simulink model "FG_traj"  (Simulink 7.8)
settings: Solver=FixedStepDiscrete  StartTime=0.0  StopTime=inf  FixedStep=Ts  RelTol=1e-3
PreLoadFcn:
  | load_waypoints
values from neighbouring files (symbols this model uses):
  g = 9.8065    [kostas_malakies.mat]    (also in kostas_malakies2.mat; load_PMModel.m = 9.81; main.m; main_last.m)
  mass = 0.66    [kostas_malakies.mat]    (also in kostas_malakies2.mat; load_PMModel.m = 0.687; main_last.m)
  pitch_cmd2pitch_1stOrd = 1.42468924998    [kostas_malakies.mat]    (also in kostas_malakies2.mat)
  roll_cmd2roll_1stOrd = 1.38101661575    [kostas_malakies.mat]    (also in kostas_malakies2.mat)
  thrust_cmd2thrust_0thOrd = 0.876575459522    [kostas_malakies.mat]    (also in kostas_malakies2.mat)
  THRUST_CMD_GAIN = -0.0835    [kostas_malakies.mat]    (also in kostas_malakies2.mat; load_PMModel.m)
  Ts = 0.02    [kostas_malakies.mat]    (also in kostas_malakies2.mat; main.m; main_last.m; matlab.mat = 0.08)
  yaw_cmd2yaw_1stOrd = 2.01792090263    [kostas_malakies.mat]    (also in kostas_malakies2.mat)
undefined symbols (not defined in the file or in its folder): DiscIntNeverNeededParam
libraries: Hquad_control_LIB_MPC x22, simulink x2
settings Model: Creator=janosch  LastModifiedBy=burrimi  SimulationMode=external
settings DataIOCC: SaveOutput=off  SaveTime=off
settings OptimizationCC: OptimizeModelRefInitCode=on  LifeSpan=Inf
settings DebuggingCC: ParameterPrecisionLossMsg=none  FcnCallInpInsideContextMsg=Use local settings
settings HardwareCC: ProdIntDivRoundTo=Zero  ProdEndianess=LittleEndian  ProdHWDeviceType=Intel Pentium
settings RTWCC: SystemTargetFile=ert.tlc  TemplateMakefile=ert_default_tmf  Description=Embedded Coder  ProcessScript=ert_make_rtw_hook  CustomHeaderCode=#include <math.h>  TargetLang=C++
settings CodeAppCC: IgnoreCustomStorageClasses=off
settings ERTTargetCC: MultiwordLength=2048  GenerateSampleERTMain=on  ExtMode=on  ERTCustomFileTemplate=example_file_process.tlc  ConvertIfToSwitch=off  SuppressUnreachableDefaultCases=off

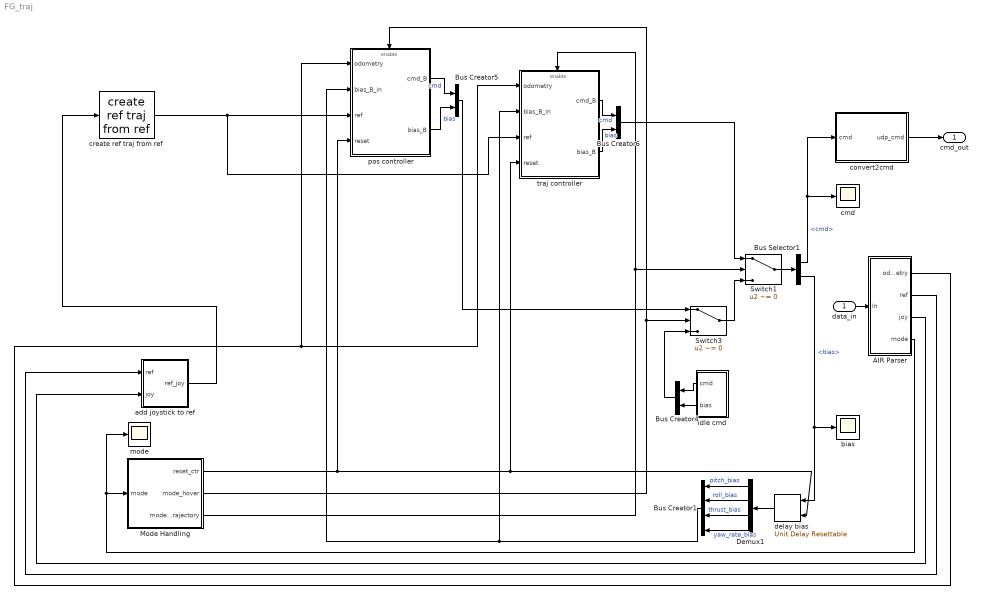
== system FG_traj ==
  data_in : Inport  OutDataTypeStr=single  PortDimensions=30
  AIR Parser : Subsystem
  Bus Creator1 : BusCreator
  Bus Creator4 : BusCreator  Inputs=2
  Bus Creator5 : BusCreator  Inputs=2
  Bus Creator6 : BusCreator  Inputs=2
  Bus Selector1 : BusSelector  OutputSignals=cmd,bias
  Demux1 : Demux
  Idle cmd : Subsystem
  Mode Handling : Subsystem
  Switch1 : Switch  Criteria=u2 ~= 0
  Switch3 : Switch  Criteria=u2 ~= 0
  add joystick to ref : Subsystem
  bias : Scope
      settings: TickLabels=on  TimeRange=40  YMin=-0.3  YMax=0.075  SaveName=ScopeData9
  cmd : Scope
      settings: YMin=-0.5  YMax=7  SaveName=ScopeData4
  convert2cmd : Subsystem
  create ref traj from ref : Hquad_control_LIB_MPC/create ref traj from ref
  delay bias : simulink/Additional Math & Discrete/Additional Discrete/Unit Delay Resettable  vinit=0.0  tsamp=-1
  mode : Scope
      settings: YMin=0  YMax=6  SaveName=ScopeData6
  pos controller : Subsystem  AncestorBlock=Hquad_control_LIB_MPC/pos controller
  traj controller : Subsystem  AncestorBlock=Hquad_control_LIB_MPC/traj controller
  cmd_out : Outport  PortDimensions=4
  wires:
  Mode Handling/1(reset_ctr) -> delay bias/2, traj controller/4(reset), pos controller/4(reset)
  Mode Handling/2(mode_hover) -> Switch3/2, pos controller/Enable
  Mode Handling/3(mode_trajectory) -> Switch1/2, traj controller/Enable
  Switch3/1 -> Switch1/3
  AIR Parser/3(joy) -> add joystick to ref/2(joy)
  add joystick to ref/1(ref_joy) -> create ref traj from ref/1
  AIR Parser/2(ref) -> add joystick to ref/1(ref)
  AIR Parser/1(odometry) -> pos controller/1(odometry), traj controller/1(odometry)
  AIR Parser/4(mode) -> Mode Handling/1(mode), mode/1
  create ref traj from ref/1 -> pos controller/3(ref), traj controller/3(ref)
  Idle cmd/1(cmd) -> Bus Creator4/1
  Idle cmd/2(bias) -> Bus Creator4/2
  Bus Creator4/1 -> Switch3/3
  traj controller/1(cmd_B) -> Bus Creator6/1  "cmd"
  traj controller/2(bias_B) -> Bus Creator6/2  "bias"
  Bus Creator6/1 -> Switch1/1
  Bus Creator5/1 -> Switch3/1
  pos controller/1(cmd_B) -> Bus Creator5/1  "cmd"
  pos controller/2(bias_B) -> Bus Creator5/2  "bias"
  Switch1/1 -> Bus Selector1/1
  Bus Selector1/1 -> cmd/1, convert2cmd/1(cmd)  "<cmd>"
  Bus Selector1/2 -> delay bias/1, bias/1  "<bias>"
  Demux1/1 -> Bus Creator1/1  "pitch_bias"
  Demux1/2 -> Bus Creator1/2  "roll_bias"
  Demux1/3 -> Bus Creator1/3  "thrust_bias"
  Demux1/4 -> Bus Creator1/4  "yaw_rate_bias"
  delay bias/1 -> Demux1/1
  Bus Creator1/1 -> pos controller/2(bias_B_in), traj controller/2(bias_B_in)
  convert2cmd/1(udp_cmd) -> cmd_out/1
  data_in/1 -> AIR Parser/1(In)

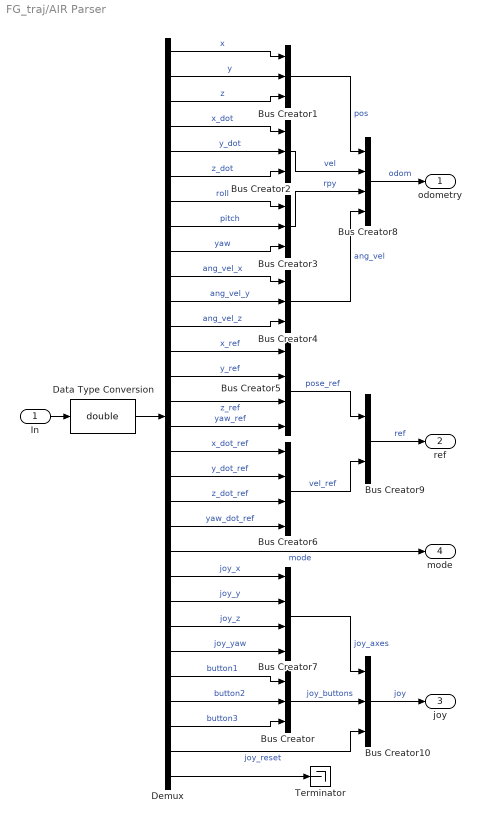
== system FG_traj/AIR Parser ==
  In : Inport
  Bus Creator{,1..4,10} (6 alike) : BusCreator  Inputs=3
  Bus Creator{5..8} (4 alike) : BusCreator
  Bus Creator9 : BusCreator  Inputs=2
  Data Type Conversion : DataTypeConversion  OutDataTypeStr=double
  Demux : Demux  Outputs=30
  Terminator : Terminator
  odometry : Outport
  ref : Outport  Port=2
  joy : Outport  Port=3
  mode : Outport  Port=4
  wires:
  In/1 -> Data Type Conversion/1
  Data Type Conversion/1 -> Demux/1
  Demux/1 -> Bus Creator1/1  "x"
  Demux/7 -> Bus Creator3/1  "roll"
  Demux/8 -> Bus Creator3/2  "pitch"
  Demux/9 -> Bus Creator3/3  "yaw"
  Demux/15 -> Bus Creator5/3  "z_ref"
  Demux/14 -> Bus Creator5/2  "y_ref"
  Demux/13 -> Bus Creator5/1  "x_ref"
  Demux/16 -> Bus Creator5/4  "yaw_ref"
  Demux/2 -> Bus Creator1/2  "y"
  Demux/3 -> Bus Creator1/3  "z"
  Demux/4 -> Bus Creator2/1  "x_dot"
  Demux/5 -> Bus Creator2/2  "y_dot"
  Demux/6 -> Bus Creator2/3  "z_dot"
  Demux/19 -> Bus Creator6/3  "z_dot_ref"
  Demux/18 -> Bus Creator6/2  "y_dot_ref"
  Demux/17 -> Bus Creator6/1  "x_dot_ref"
  Demux/20 -> Bus Creator6/4  "yaw_dot_ref"
  Demux/12 -> Bus Creator4/3  "ang_vel_z"
  Demux/11 -> Bus Creator4/2  "ang_vel_y"
  Demux/10 -> Bus Creator4/1  "ang_vel_x"
  Demux/21 -> mode/1  "mode"
  Bus Creator5/1 -> Bus Creator9/1  "pose_ref"
  Bus Creator6/1 -> Bus Creator9/2  "vel_ref"
  Demux/22 -> Bus Creator7/1  "joy_x"
  Demux/23 -> Bus Creator7/2  "joy_y"
  Demux/24 -> Bus Creator7/3  "joy_z"
  Demux/25 -> Bus Creator7/4  "joy_yaw"
  Bus Creator7/1 -> Bus Creator10/1  "joy_axes"
  Demux/26 -> Bus Creator/1  "button1"
  Demux/28 -> Bus Creator/3  "button3"
  Demux/27 -> Bus Creator/2  "button2"
  Bus Creator/1 -> Bus Creator10/2  "joy_buttons"
  Bus Creator4/1 -> Bus Creator8/4  "ang_vel"
  Bus Creator3/1 -> Bus Creator8/3  "rpy"
  Bus Creator2/1 -> Bus Creator8/2  "vel"
  Bus Creator1/1 -> Bus Creator8/1  "pos"
  Demux/29 -> Bus Creator10/3  "joy_reset"
  Bus Creator10/1 -> joy/1  "joy"
  Bus Creator9/1 -> ref/1  "ref"
  Bus Creator8/1 -> odometry/1  "odom"
  Demux/30 -> Terminator/1

== system FG_traj/Idle cmd ==
  Bus Creator : BusCreator
  Bus Creator3 : BusCreator
  pitch : Constant  Value=0
  pitch_bias : Constant  Value=0
  roll : Constant  Value=0
  roll_bias : Constant  Value=0
  thrust : Constant  Value=-mass*g
  thrust_bias : Constant  Value=0
  yaw : Constant  Value=0
  yaw_rate_bias : Constant  Value=0
  cmd : Outport
  bias : Outport  Port=2
  wires:
  roll/1 -> Bus Creator/2  "roll_cmd"
  pitch/1 -> Bus Creator/1  "pitch_cmd"
  Bus Creator/1 -> cmd/1  "cmd"
  thrust/1 -> Bus Creator/3  "thrust_cmd"
  yaw/1 -> Bus Creator/4  "yaw_rate_cmd"
  pitch_bias/1 -> Bus Creator3/1  "pitch_bias"
  roll_bias/1 -> Bus Creator3/2  "roll_bias"
  thrust_bias/1 -> Bus Creator3/3  "thrust_bias"
  yaw_rate_bias/1 -> Bus Creator3/4  "yaw_rate_bias"
  Bus Creator3/1 -> bias/1  "bias"

== system FG_traj/Mode Handling ==
  mode : Inport
  Constant1 : Constant
  Constant2 : Constant  Value=0
  Multiport Switch : MultiPortSwitch  DataPortOrder=Specify indices  Inputs=2  DataPortIndices={[1,2,3],0}  zeroidx=off
  Multiport Switch1 : MultiPortSwitch  DataPortOrder=Specify indices  Inputs=2  DataPortIndices={[10],0}  zeroidx=off
  Multiport Switch2 : MultiPortSwitch  DataPortOrder=Specify indices  Inputs=2  DataPortIndices={[4],0}  zeroidx=off
  reset_ctr : Outport
  mode_hover : Outport  Port=2
  mode_trajectory : Outport  Port=3
  wires:
  Constant1/1 -> Multiport Switch/2, Multiport Switch1/2, Multiport Switch2/2
  Constant2/1 -> Multiport Switch/3, Multiport Switch1/3, Multiport Switch2/3
  Multiport Switch1/1 -> reset_ctr/1
  mode/1 -> Multiport Switch/1, Multiport Switch1/1, Multiport Switch2/1
  Multiport Switch/1 -> mode_hover/1
  Multiport Switch2/1 -> mode_trajectory/1

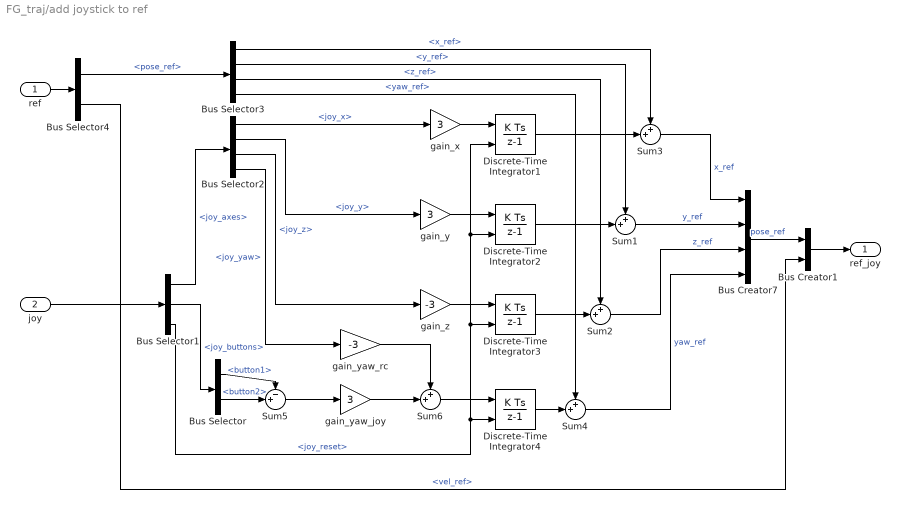
== system FG_traj/add joystick to ref ==
  ref : Inport
  joy : Inport  Port=2
  Bus Creator1 : BusCreator  Inputs=2
  Bus Creator7 : BusCreator
  Bus Selector : BusSelector  OutputSignals=button1,button2
  Bus Selector1 : BusSelector  OutputSignals=joy_axes,joy_buttons,joy_reset
  Bus Selector2 : BusSelector  OutputSignals=joy_x,joy_y,joy_z,joy_yaw
  Bus Selector3 : BusSelector  OutputSignals=x_ref,y_ref,z_ref,yaw_ref
  Bus Selector4 : BusSelector  OutputSignals=pose_ref,vel_ref
  Discrete-Time Integrator{1..4} (4 alike) : DiscreteIntegrator  ExternalReset=rising  SampleTime=Ts  ICPrevOutput=DiscIntNeverNeededParam  ICPrevScaledInput=DiscIntNeverNeededParam
  Sum{1..4,6} (5 alike) : Sum  Inputs=++|
  Sum5 : Sum  Inputs=-+|
  gain_x : Gain  Gain=3
  gain_y : Gain  Gain=3
  gain_yaw_joy : Gain  Gain=3
  gain_yaw_rc : Gain  Gain=-3
  gain_z : Gain  Gain=-3
  ref_joy : Outport
  wires:
  Bus Selector2/1 -> gain_x/1  "<joy_x>"
  Bus Selector2/2 -> gain_y/1  "<joy_y>"
  Bus Selector2/3 -> gain_z/1  "<joy_z>"
  gain_x/1 -> Discrete-Time Integrator1/1
  gain_y/1 -> Discrete-Time Integrator2/1
  gain_z/1 -> Discrete-Time Integrator3/1
  Bus Selector3/1 -> Sum3/1  "<x_ref>"
  Bus Selector3/2 -> Sum1/1  "<y_ref>"
  Bus Selector3/3 -> Sum2/1  "<z_ref>"
  Discrete-Time Integrator1/1 -> Sum3/2
  Discrete-Time Integrator2/1 -> Sum1/2
  Discrete-Time Integrator3/1 -> Sum2/2
  Sum4/1 -> Bus Creator7/4  "yaw_ref"
  Sum2/1 -> Bus Creator7/3  "z_ref"
  Sum1/1 -> Bus Creator7/2  "y_ref"
  Sum3/1 -> Bus Creator7/1  "x_ref"
  Bus Selector1/2 -> Bus Selector/1  "<joy_buttons>"
  Bus Selector1/3 -> Discrete-Time Integrator3/2, Discrete-Time Integrator1/2, Discrete-Time Integrator2/2, Discrete-Time Integrator4/2  "<joy_reset>"
  Bus Selector/1 -> Sum5/1  "<button1>"
  Bus Selector/2 -> Sum5/2  "<button2>"
  Discrete-Time Integrator4/1 -> Sum4/2
  Bus Selector3/4 -> Sum4/1  "<yaw_ref>"
  joy/1 -> Bus Selector1/1
  Bus Selector1/1 -> Bus Selector2/1  "<joy_axes>"
  ref/1 -> Bus Selector4/1
  Bus Creator1/1 -> ref_joy/1
  Sum5/1 -> gain_yaw_joy/1
  Sum6/1 -> Discrete-Time Integrator4/1
  Bus Selector2/4 -> gain_yaw_rc/1  "<joy_yaw>"
  gain_yaw_rc/1 -> Sum6/1
  gain_yaw_joy/1 -> Sum6/2
  Bus Creator7/1 -> Bus Creator1/1  "pose_ref"
  Bus Selector4/1 -> Bus Selector3/1  "<pose_ref>"
  Bus Selector4/2 -> Bus Creator1/2  "<vel_ref>"

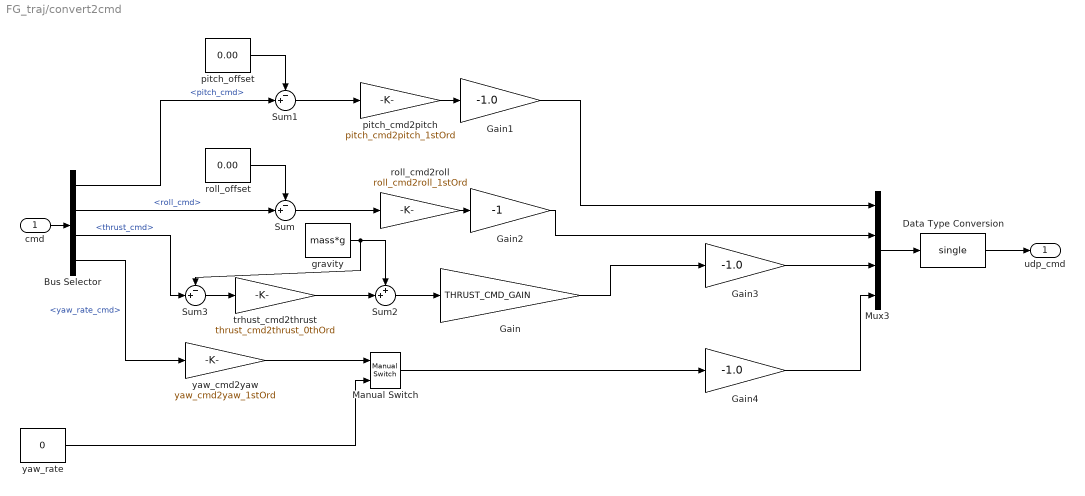
== system FG_traj/convert2cmd ==
  cmd : Inport
  Bus Selector : BusSelector  OutputSignals=pitch_cmd,roll_cmd,thrust_cmd,yaw_rate_cmd
  Data Type Conversion : DataTypeConversion  OutDataTypeStr=single
  Gain : Gain  Gain=THRUST_CMD_GAIN
  Gain1 : Gain  Gain=-1.0
  Gain2 : Gain  Gain=-1
  Gain3 : Gain  Gain=-1.0
  Gain4 : Gain  Gain=-1.0
  Manual Switch : simulink/Signal Routing/Manual Switch  sw=1  action=0  varsize=off
  Mux3 : Mux
  Sum : Sum  Inputs=-+|
  Sum1 : Sum  Inputs=-+|
  Sum2 : Sum  Inputs=++|
  Sum3 : Sum  Inputs=-+|
  gravity : Constant  Value=mass*g
  pitch_cmd2pitch : Gain  Gain=pitch_cmd2pitch_1stOrd
  pitch_offset : Constant  Value=0.00
  roll_cmd2roll : Gain  Gain=roll_cmd2roll_1stOrd
  roll_offset : Constant  Value=0.00
  trhust_cmd2thrust : Gain  Gain=thrust_cmd2thrust_0thOrd
  yaw_cmd2yaw : Gain  Gain=yaw_cmd2yaw_1stOrd
  yaw_rate : Constant  Value=0
  udp_cmd : Outport
  wires:
  pitch_cmd2pitch/1 -> Gain1/1
  Bus Selector/2 -> Sum/2  "<roll_cmd>"
  Sum/1 -> roll_cmd2roll/1
  roll_offset/1 -> Sum/1
  Gain4/1 -> Mux3/4
  Gain3/1 -> Mux3/3
  Gain2/1 -> Mux3/2
  Gain/1 -> Gain3/1
  Gain1/1 -> Mux3/1
  pitch_offset/1 -> Sum1/1
  Sum1/1 -> pitch_cmd2pitch/1
  Mux3/1 -> Data Type Conversion/1
  Data Type Conversion/1 -> udp_cmd/1
  gravity/1 -> Sum2/1, Sum3/1
  Sum2/1 -> Gain/1
  Manual Switch/1 -> Gain4/1
  yaw_rate/1 -> Manual Switch/2
  cmd/1 -> Bus Selector/1
  Bus Selector/1 -> Sum1/2  "<pitch_cmd>"
  yaw_cmd2yaw/1 -> Manual Switch/1
  trhust_cmd2thrust/1 -> Sum2/2
  roll_cmd2roll/1 -> Gain2/1
  Bus Selector/3 -> Sum3/2  "<thrust_cmd>"
  Sum3/1 -> trhust_cmd2thrust/1
  Bus Selector/4 -> yaw_cmd2yaw/1  "<yaw_rate_cmd>"

== system FG_traj/pos controller ==
  odometry : Inport
  bias_B_in : Inport  Port=2
  ref : Inport  Port=3
  reset : Inport  Port=4
  Enable : EnablePort  StatesWhenEnabling=reset
  MAIN CONTROL LOOP1 : Subsystem  Priority=2  AncestorBlock=Hquad_control_LIB_MPC/MAIN CONTROL LOOP  TreatAsAtomicUnit=on
  decoupling and rotation : Hquad_control_LIB_MPC/decoupling and rotation  Priority=3
  get ref from vector : Subsystem
  rotate to world frame : Hquad_control_LIB_MPC/rotate to world frame  Priority=1
  view & log signals : Subsystem  AncestorBlock=Hquad_control_LIB_MPC/view & log signals
  cmd_B : Outport
  bias_B : Outport  Port=2
  wires:
  MAIN CONTROL LOOP1/1(cmd_W) -> decoupling and rotation/2, view & log signals/3(cmd)
  odometry/1 -> rotate to world frame/1, view & log signals/1(odometry)
  reset/1 -> MAIN CONTROL LOOP1/4(reset)
  ref/1 -> get ref from vector/1(X_ref), MAIN CONTROL LOOP1/3(ref)
  get ref from vector/1(ref) -> view & log signals/2(ref)
  rotate to world frame/1 -> MAIN CONTROL LOOP1/1(odometry), decoupling and rotation/1
  MAIN CONTROL LOOP1/2(bias_W_out) -> decoupling and rotation/3, view & log signals/4(bias)
  decoupling and rotation/1 -> cmd_B/1
  decoupling and rotation/2 -> bias_B/1
  rotate to world frame/2 -> MAIN CONTROL LOOP1/2(bias_W)
  bias_B_in/1 -> rotate to world frame/2

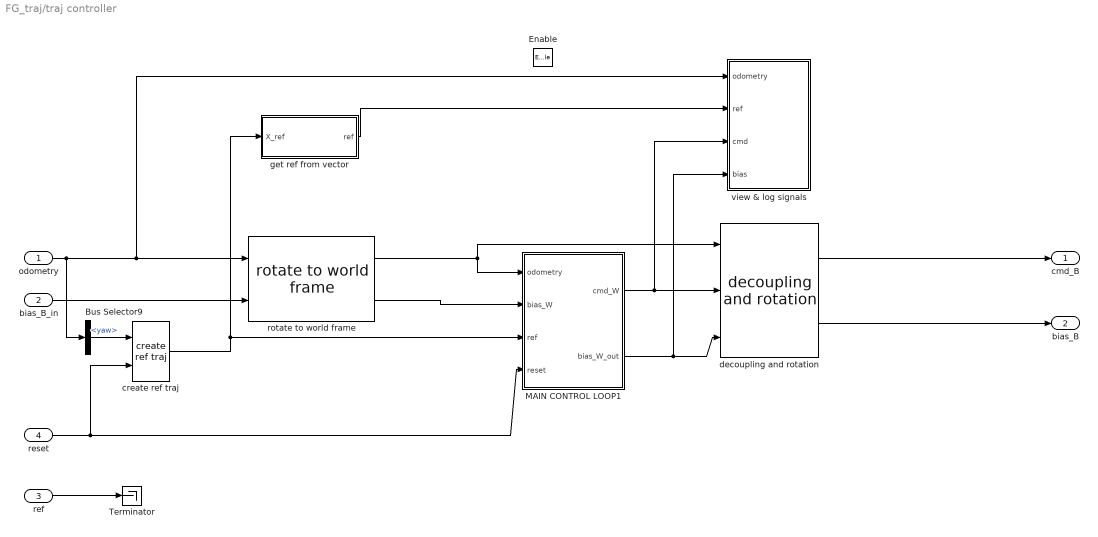
== system FG_traj/traj controller ==
  odometry : Inport
  bias_B_in : Inport  Port=2
  ref : Inport  Port=3
  reset : Inport  Port=4
  Enable : EnablePort  StatesWhenEnabling=reset
  Bus Selector9 : BusSelector  OutputSignals=rpy.yaw
  MAIN CONTROL LOOP1 : Subsystem  Priority=2  AncestorBlock=Hquad_control_LIB_MPC/MAIN CONTROL LOOP  TreatAsAtomicUnit=on
  Terminator : Terminator
  create ref traj : Hquad_control_LIB_MPC/create ref traj
  decoupling and rotation : Hquad_control_LIB_MPC/decoupling and rotation  Priority=3
  get ref from vector : Subsystem
  rotate to world frame : Hquad_control_LIB_MPC/rotate to world frame  Priority=1
  view & log signals : Subsystem  AncestorBlock=Hquad_control_LIB_MPC/view & log signals
  cmd_B : Outport
  bias_B : Outport  Port=2
  wires:
  ref/1 -> Terminator/1
  Bus Selector9/1 -> create ref traj/1  "<yaw>"
  bias_B_in/1 -> rotate to world frame/2
  rotate to world frame/2 -> MAIN CONTROL LOOP1/2(bias_W)
  decoupling and rotation/2 -> bias_B/1
  decoupling and rotation/1 -> cmd_B/1
  MAIN CONTROL LOOP1/2(bias_W_out) -> decoupling and rotation/3, view & log signals/4(bias)
  rotate to world frame/1 -> decoupling and rotation/1, MAIN CONTROL LOOP1/1(odometry)
  get ref from vector/1(ref) -> view & log signals/2(ref)
  reset/1 -> create ref traj/2, MAIN CONTROL LOOP1/4(reset)
  odometry/1 -> rotate to world frame/1, view & log signals/1(odometry), Bus Selector9/1
  MAIN CONTROL LOOP1/1(cmd_W) -> decoupling and rotation/2, view & log signals/3(cmd)
  create ref traj/1 -> get ref from vector/1(X_ref), MAIN CONTROL LOOP1/3(ref)

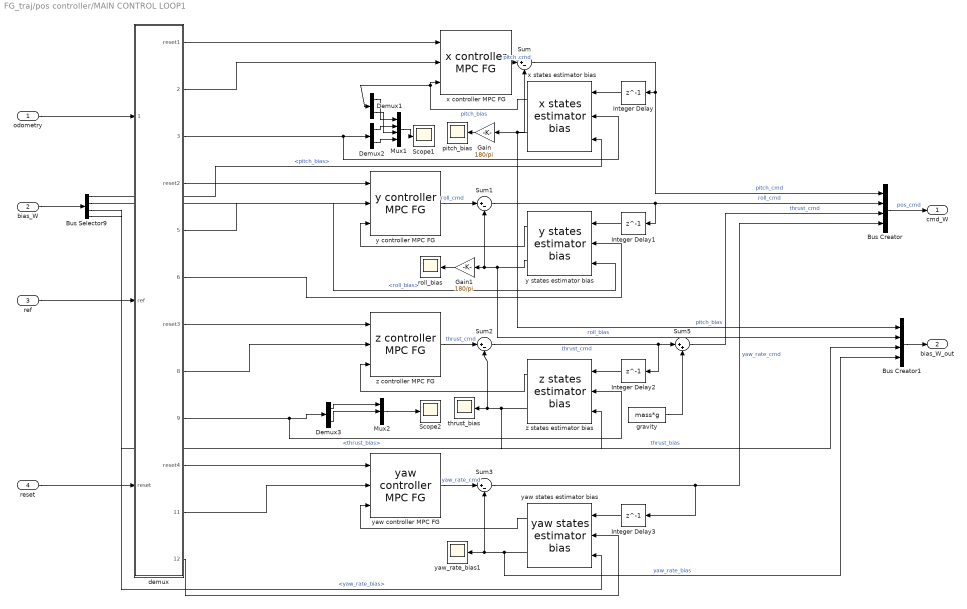
== system FG_traj/pos controller/MAIN CONTROL LOOP1 ==
  odometry : Inport
  bias_W : Inport  Port=2
  ref : Inport  Port=3
  reset : Inport  Port=4
  Bus Creator : BusCreator
  Bus Creator1 : BusCreator
  Bus Selector9 : BusSelector  OutputSignals=pitch_bias,roll_bias,thrust_bias,yaw_rate_bias
  Demux1 : Demux  Outputs=3
  Demux2 : Demux  Outputs=3
  Demux3 : Demux  Outputs=2
  Gain : Gain  Gain=180/pi
  Gain1 : Gain  Gain=180/pi
  Integer Delay{,1..3} (4 alike) : Delay  DelayLength=1
  Mux1 : Mux
  Mux2 : Mux  Inputs=5
  Scope1 : Scope
      settings: YMin=-0.05  YMax=1.05  SaveName=ScopeData6
  Scope2 : Scope
      settings: YMin=-0.4  YMax=1.4  SaveName=ScopeData15
  Sum{,1..3} (4 alike) : Sum  Inputs=|+-
  Sum5 : Sum  Inputs=|++
  demux : Subsystem
  gravity : Constant  Value=mass*g
  pitch_bias : Scope
      settings: YMin=0  YMax=3.75  SaveName=ScopeData7
  roll_bias : Scope
      settings: YMin=-1  YMax=1  SaveName=ScopeData12
  thrust_bias : Scope
      settings: YMin=0  YMax=0.3  SaveName=ScopeData13
  "x controller MPC FG  " : Hquad_control_LIB_MPC/x controller MPC FG  
  x states estimator bias : Hquad_control_LIB_MPC/x states estimator bias
  y controller MPC FG : Hquad_control_LIB_MPC/y controller MPC FG
  y states estimator bias : Hquad_control_LIB_MPC/y states estimator bias
  yaw controller MPC FG : Hquad_control_LIB_MPC/yaw controller MPC FG
  yaw states estimator bias : Hquad_control_LIB_MPC/yaw states estimator bias
  yaw_rate_bias1 : Scope
      settings: YMin=-1  YMax=1  SaveName=ScopeData16
  z controller MPC FG : Hquad_control_LIB_MPC/z controller MPC FG
  z states estimator bias : Hquad_control_LIB_MPC/z states estimator bias
  cmd_W : Outport
  bias_W_out : Outport  Port=2
  wires:
  Bus Selector9/4 -> yaw states estimator bias/3  "<yaw_rate_bias>"
  Sum3/1 -> Integer Delay3/1, Bus Creator/4  "yaw_rate_cmd"
  yaw controller MPC FG/1 -> Sum3/1  "yaw_rate_cmd"
  yaw states estimator bias/2 -> Bus Creator1/4, Sum3/2, yaw_rate_bias1/1  "yaw_rate_bias"
  yaw states estimator bias/1 -> yaw controller MPC FG/3
  Integer Delay3/1 -> yaw states estimator bias/1
  Bus Selector9/3 -> z states estimator bias/3  "<thrust_bias>"
  x states estimator bias/2 -> Sum/2, Bus Creator1/1, Gain/1  "pitch_bias"
  Demux2/3 -> Mux1/4
  Demux1/3 -> Mux1/3
  x states estimator bias/1 -> "x controller MPC FG  "/3, Demux1/1  "pitch_bias"
  demux/12(yaw_states_meas) -> yaw states estimator bias/2
  Gain1/1 -> roll_bias/1
  Gain/1 -> pitch_bias/1
  Bus Selector9/1 -> x states estimator bias/3  "<pitch_bias>"
  Bus Selector9/2 -> y states estimator bias/3  "<roll_bias>"
  bias_W/1 -> Bus Selector9/1
  Sum5/1 -> Bus Creator/3  "thrust_cmd"
  gravity/1 -> Sum5/2
  Bus Creator1/1 -> bias_W_out/1
  Sum2/1 -> Sum5/1, Integer Delay2/1  "thrust_cmd"
  z controller MPC FG/1 -> Sum2/1  "thrust_cmd"
  z states estimator bias/2 -> Sum2/2, thrust_bias/1, Bus Creator1/3  "thrust_bias"
  y states estimator bias/2 -> Bus Creator1/2, Sum1/2, Gain1/1  "roll_bias"
  Sum1/1 -> Bus Creator/2, Integer Delay1/1  "roll_cmd"
  y controller MPC FG/1 -> Sum1/1  "roll_cmd"
  Sum/1 -> Bus Creator/1, Integer Delay/1  "pitch_cmd"
  "x controller MPC FG  "/1 -> Sum/1  "pitch_cmd"
  Mux1/1 -> Scope1/1
  Demux2/1 -> Mux1/2
  Demux1/1 -> Mux1/1
  y states estimator bias/1 -> y controller MPC FG/3
  Integer Delay/1 -> x states estimator bias/1
  Demux3/2 -> Mux2/3
  Demux3/1 -> Mux2/1
  Mux2/1 -> Scope2/1
  z states estimator bias/1 -> z controller MPC FG/3
  demux/8(X_ref_z) -> z controller MPC FG/2
  demux/2(X_ref_x) -> "x controller MPC FG  "/2
  Integer Delay1/1 -> y states estimator bias/1
  Integer Delay2/1 -> z states estimator bias/1
  odometry/1 -> demux/1(odometry)
  ref/1 -> demux/2(ref)
  reset/1 -> demux/3(reset)
  demux/1(reset1) -> "x controller MPC FG  "/1
  demux/4(reset2) -> y controller MPC FG/1
  demux/5(X_ref_y) -> y controller MPC FG/2
  demux/7(reset3) -> z controller MPC FG/1
  demux/10(reset4) -> yaw controller MPC FG/1
  Bus Creator/1 -> cmd_W/1  "pos_cmd"
  demux/3(x_states_meas) -> x states estimator bias/2, Demux2/1
  demux/6(y_states_meas) -> y states estimator bias/2
  demux/9(z_states_meas) -> z states estimator bias/2, Demux3/1
  demux/11(X_ref_yaw) -> yaw controller MPC FG/2

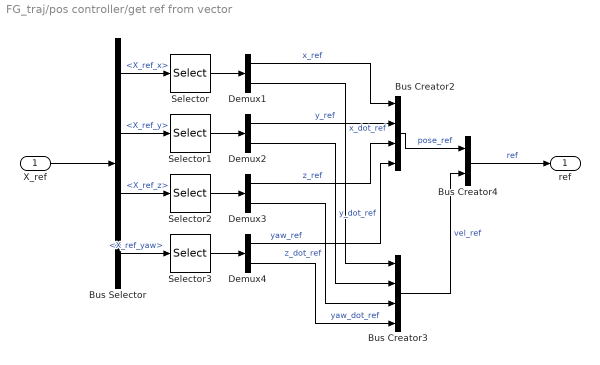
== system FG_traj/pos controller/get ref from vector ==
  X_ref : Inport
  Bus Creator2 : BusCreator
  Bus Creator3 : BusCreator
  Bus Creator4 : BusCreator  Inputs=2
  Bus Selector : BusSelector  OutputSignals=X_ref_x,X_ref_y,X_ref_z,X_ref_yaw
  Demux{1..4} (4 alike) : Demux  Outputs=2
  Selector{,1..3} (4 alike) : Selector  IndexOptions=Index vector (dialog)  Indices=[1 2]  OutputSizes=1
  ref : Outport
  wires:
  X_ref/1 -> Bus Selector/1
  Bus Selector/1 -> Selector/1  "<X_ref_x>"
  Bus Selector/4 -> Selector3/1  "<X_ref_yaw>"
  Bus Selector/3 -> Selector2/1  "<X_ref_z>"
  Bus Selector/2 -> Selector1/1  "<X_ref_y>"
  Selector/1 -> Demux1/1
  Selector3/1 -> Demux4/1
  Selector2/1 -> Demux3/1
  Selector1/1 -> Demux2/1
  Bus Creator2/1 -> Bus Creator4/1  "pose_ref"
  Bus Creator3/1 -> Bus Creator4/2  "vel_ref"
  Bus Creator4/1 -> ref/1  "ref"
  Demux1/1 -> Bus Creator2/1  "x_ref"
  Demux2/1 -> Bus Creator2/2  "y_ref"
  Demux3/1 -> Bus Creator2/3  "z_ref"
  Demux4/1 -> Bus Creator2/4  "yaw_ref"
  Demux1/2 -> Bus Creator3/1  "x_dot_ref"
  Demux2/2 -> Bus Creator3/2  "y_dot_ref"
  Demux3/2 -> Bus Creator3/3  "z_dot_ref"
  Demux4/2 -> Bus Creator3/4  "yaw_dot_ref"

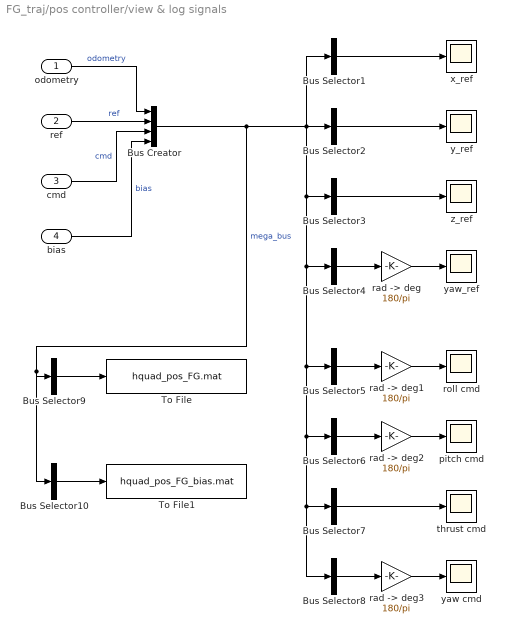
== system FG_traj/pos controller/view & log signals ==
  odometry : Inport
  ref : Inport  Port=2
  cmd : Inport  Port=3
  bias : Inport  Port=4
  Bus Creator : BusCreator
  Bus Selector1 : BusSelector  OutputSignals=odometry.pos.x,odometry.vel.x_dot,ref.pose_ref.x_ref,ref.vel_ref.x_dot_ref  OutputAsBus=on
  Bus Selector10 : BusSelector  OutputSignals=bias.pitch_bias,bias.roll_bias,bias.thrust_bias,bias.yaw_rate_bias  OutputAsBus=on
  Bus Selector2 : BusSelector  OutputSignals=odometry.pos.y,odometry.vel.y_dot,ref.pose_ref.y_ref,ref.vel_ref.y_dot_ref  OutputAsBus=on
  Bus Selector3 : BusSelector  OutputSignals=odometry.pos.z,odometry.vel.z_dot,ref.pose_ref.z_ref,ref.vel_ref.z_dot_ref  OutputAsBus=on
  Bus Selector4 : BusSelector  OutputSignals=odometry.rpy.yaw,odometry.ang_vel.ang_vel_z,ref.pose_ref.yaw_ref,ref.vel_ref.yaw_dot_ref  OutputAsBus=on
  Bus Selector5 : BusSelector  OutputSignals=odometry.rpy.roll,odometry.ang_vel.ang_vel_x,cmd.roll_cmd  OutputAsBus=on
  Bus Selector6 : BusSelector  OutputSignals=odometry.rpy.pitch,odometry.ang_vel.ang_vel_y,cmd.pitch_cmd  OutputAsBus=on
  Bus Selector7 : BusSelector  OutputSignals=odometry.pos.z,ref.pose_ref.z_ref,cmd.thrust_cmd  OutputAsBus=on
  Bus Selector8 : BusSelector  OutputSignals=odometry.rpy.yaw,odometry.ang_vel.ang_vel_z,cmd.yaw_rate_cmd  OutputAsBus=on
  Bus Selector9 : BusSelector  OutputSignals=odometry.pos.x,odometry.vel.x_dot,odometry.rpy.pitch,ref.pose_ref.x_ref,cmd.pitch_cmd,odometry.pos.y,odometry.vel.y_dot,odometry.rpy.roll,ref.pose_ref.y_ref,cmd.roll_cmd,odometry.pos.z,odometry.vel.z_dot,ref.pose_ref.z_ref,cmd.thrust_cmd,odometry.rpy.yaw,odometry.ang_vel.ang_vel_z,ref.pose_ref.yaw_ref,cmd.yaw_rate_cmd  OutputAsBus=on
  To File : ToFile  Filename=hquad_pos_FG.mat  MatrixName=hquad_pos_FG
  To File1 : ToFile  Filename=hquad_pos_FG_bias.mat  MatrixName=hquad_pos_FG_bias
  pitch cmd : Scope
      settings: YMin=-15  YMax=15  SaveName=ScopeData2
  rad -> deg{,1..3} (4 alike) : Gain  Gain=180/pi
  roll cmd : Scope
      settings: YMin=-100  YMax=100
  thrust cmd : Scope
      settings: YMin=-3  YMax=3  SaveName=ScopeData11
  x_ref : Scope
      settings: TimeRange=40  YMin=-1.5  YMax=1.5  SaveName=ScopeData3
  y_ref : Scope
      settings: TimeRange=40  YMin=-0.75  YMax=2.75
  yaw cmd : Scope
      settings: YMin=-60  YMax=60  SaveName=ScopeData10
  yaw_ref : Scope
      settings: TimeRange=39.996  YMin=-190  YMax=190  SaveName=ScopeData8
  z_ref : Scope
      settings: TimeRange=40  YMin=-21  YMax=1  SaveName=ScopeData5
  wires:
  Bus Selector10/1 -> To File1/1
  bias/1 -> Bus Creator/4  "bias"
  Bus Selector8/1 -> "rad -> deg3"/1
  Bus Selector6/1 -> "rad -> deg2"/1
  Bus Selector5/1 -> "rad -> deg1"/1
  Bus Selector7/1 -> thrust cmd/1
  Bus Selector4/1 -> "rad -> deg"/1
  Bus Selector3/1 -> z_ref/1
  Bus Selector2/1 -> y_ref/1
  Bus Selector1/1 -> x_ref/1
  Bus Creator/1 -> Bus Selector10/1, Bus Selector9/1, Bus Selector8/1, Bus Selector7/1, Bus Selector6/1, Bus Selector5/1, Bus Selector4/1, Bus Selector3/1, Bus Selector2/1, Bus Selector1/1  "mega_bus"
  cmd/1 -> Bus Creator/3  "cmd"
  ref/1 -> Bus Creator/2  "ref"
  odometry/1 -> Bus Creator/1  "odometry"
  "rad -> deg3"/1 -> yaw cmd/1
  "rad -> deg2"/1 -> pitch cmd/1
  "rad -> deg1"/1 -> roll cmd/1
  "rad -> deg"/1 -> yaw_ref/1
  Bus Selector9/1 -> To File/1

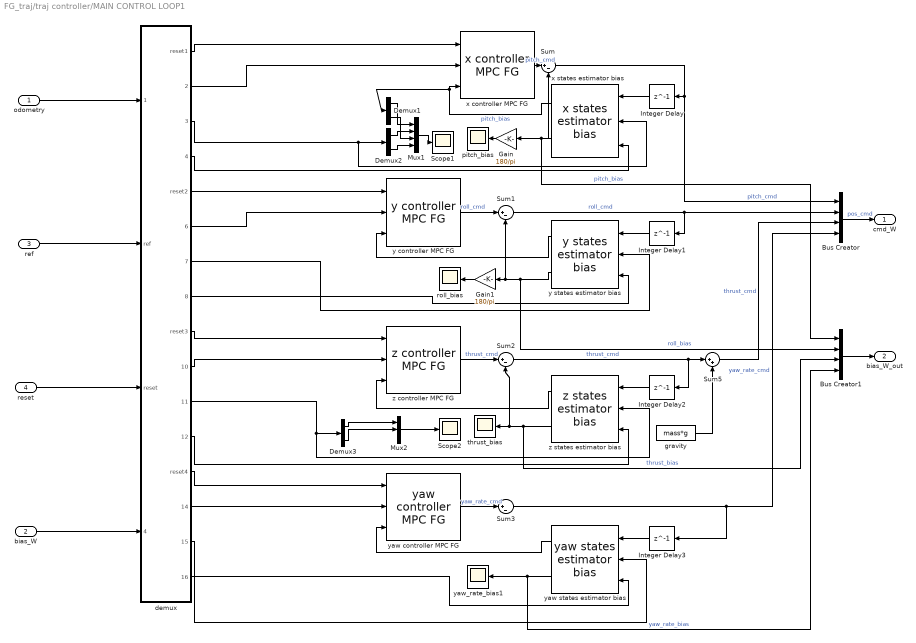
== system FG_traj/traj controller/MAIN CONTROL LOOP1 ==
  odometry : Inport
  bias_W : Inport  Port=2
  ref : Inport  Port=3
  reset : Inport  Port=4
  Bus Creator : BusCreator
  Bus Creator1 : BusCreator
  Demux1 : Demux  Outputs=3
  Demux2 : Demux  Outputs=3
  Demux3 : Demux  Outputs=2
  Gain : Gain  Gain=180/pi
  Gain1 : Gain  Gain=180/pi
  Integer Delay{,1..3} (4 alike) : Delay  DelayLength=1
  Mux1 : Mux
  Mux2 : Mux  Inputs=5
  Scope1 : Scope
      settings: YMin=-0.05  YMax=1.05  SaveName=ScopeData6
  Scope2 : Scope
      settings: YMin=-0.4  YMax=1.4  SaveName=ScopeData15
  Sum{,1..3} (4 alike) : Sum  Inputs=|+-
  Sum5 : Sum  Inputs=|++
  demux : Subsystem
  gravity : Constant  Value=mass*g
  pitch_bias : Scope
      settings: YMin=0  YMax=3.75  SaveName=ScopeData7
  roll_bias : Scope
      settings: YMin=-1  YMax=1  SaveName=ScopeData12
  thrust_bias : Scope
      settings: YMin=0  YMax=0.3  SaveName=ScopeData13
  "x controller MPC FG  " : Hquad_control_LIB_MPC/x controller MPC FG  
  x states estimator bias : Hquad_control_LIB_MPC/x states estimator bias
  y controller MPC FG : Hquad_control_LIB_MPC/y controller MPC FG
  y states estimator bias : Hquad_control_LIB_MPC/y states estimator bias
  yaw controller MPC FG : Hquad_control_LIB_MPC/yaw controller MPC FG
  yaw states estimator bias : Hquad_control_LIB_MPC/yaw states estimator bias
  yaw_rate_bias1 : Scope
      settings: YMin=-1  YMax=1  SaveName=ScopeData16
  z controller MPC FG : Hquad_control_LIB_MPC/z controller MPC FG
  z states estimator bias : Hquad_control_LIB_MPC/z states estimator bias
  cmd_W : Outport
  bias_W_out : Outport  Port=2
  wires:
  demux/4(pitch_bias) -> x states estimator bias/3
  demux/8(roll_bias) -> y states estimator bias/3
  demux/12(thrust_bias) -> z states estimator bias/3
  demux/16(yaw_rate_bias) -> yaw states estimator bias/3
  bias_W/1 -> demux/4(bias_W)
  Sum3/1 -> Integer Delay3/1, Bus Creator/4  "yaw_rate_cmd"
  yaw controller MPC FG/1 -> Sum3/1  "yaw_rate_cmd"
  yaw states estimator bias/2 -> Bus Creator1/4, yaw_rate_bias1/1  "yaw_rate_bias"
  yaw states estimator bias/1 -> yaw controller MPC FG/3
  Integer Delay3/1 -> yaw states estimator bias/1
  x states estimator bias/2 -> Sum/2, Bus Creator1/1, Gain/1  "pitch_bias"
  Demux2/3 -> Mux1/4
  Demux1/3 -> Mux1/3
  x states estimator bias/1 -> "x controller MPC FG  "/3, Demux1/1  "pitch_bias"
  demux/15(yaw_states_meas) -> yaw states estimator bias/2
  Gain1/1 -> roll_bias/1
  Gain/1 -> pitch_bias/1
  Sum5/1 -> Bus Creator/3  "thrust_cmd"
  gravity/1 -> Sum5/2
  Bus Creator1/1 -> bias_W_out/1
  Sum2/1 -> Sum5/1, Integer Delay2/1  "thrust_cmd"
  z controller MPC FG/1 -> Sum2/1  "thrust_cmd"
  z states estimator bias/2 -> Sum2/2, thrust_bias/1, Bus Creator1/3  "thrust_bias"
  y states estimator bias/2 -> Bus Creator1/2, Sum1/2, Gain1/1  "roll_bias"
  Sum1/1 -> Bus Creator/2, Integer Delay1/1  "roll_cmd"
  y controller MPC FG/1 -> Sum1/1  "roll_cmd"
  Sum/1 -> Bus Creator/1, Integer Delay/1  "pitch_cmd"
  "x controller MPC FG  "/1 -> Sum/1  "pitch_cmd"
  Mux1/1 -> Scope1/1
  Demux2/1 -> Mux1/2
  Demux1/1 -> Mux1/1
  y states estimator bias/1 -> y controller MPC FG/3
  Integer Delay/1 -> x states estimator bias/1
  Demux3/2 -> Mux2/3
  Demux3/1 -> Mux2/1
  Mux2/1 -> Scope2/1
  z states estimator bias/1 -> z controller MPC FG/3
  demux/10(X_ref_z) -> z controller MPC FG/2
  demux/2(X_ref_x) -> "x controller MPC FG  "/2
  Integer Delay1/1 -> y states estimator bias/1
  Integer Delay2/1 -> z states estimator bias/1
  odometry/1 -> demux/1(odometry)
  ref/1 -> demux/2(ref)
  reset/1 -> demux/3(reset)
  demux/1(reset1) -> "x controller MPC FG  "/1
  demux/5(reset2) -> y controller MPC FG/1
  demux/6(X_ref_y) -> y controller MPC FG/2
  demux/9(reset3) -> z controller MPC FG/1
  demux/13(reset4) -> yaw controller MPC FG/1
  Bus Creator/1 -> cmd_W/1  "pos_cmd"
  demux/3(x_states_meas) -> x states estimator bias/2, Demux2/1
  demux/7(y_states_meas) -> y states estimator bias/2
  demux/11(z_states_meas) -> z states estimator bias/2, Demux3/1
  demux/14(X_ref_yaw) -> yaw controller MPC FG/2

== system FG_traj/traj controller/get ref from vector ==
  X_ref : Inport
  Bus Creator2 : BusCreator
  Bus Creator3 : BusCreator
  Bus Creator4 : BusCreator  Inputs=2
  Bus Selector : BusSelector  OutputSignals=X_ref_x,X_ref_y,X_ref_z,X_ref_yaw
  Demux{1..4} (4 alike) : Demux  Outputs=2
  Selector{,1..3} (4 alike) : Selector  IndexOptions=Index vector (dialog)  Indices=[1 2]  OutputSizes=1
  ref : Outport
  wires:
  Demux4/2 -> Bus Creator3/4  "yaw_dot_ref"
  Demux3/2 -> Bus Creator3/3  "z_dot_ref"
  Demux2/2 -> Bus Creator3/2  "y_dot_ref"
  Demux1/2 -> Bus Creator3/1  "x_dot_ref"
  Demux4/1 -> Bus Creator2/4  "yaw_ref"
  Demux3/1 -> Bus Creator2/3  "z_ref"
  Demux2/1 -> Bus Creator2/2  "y_ref"
  Demux1/1 -> Bus Creator2/1  "x_ref"
  Bus Creator4/1 -> ref/1  "ref"
  Bus Creator3/1 -> Bus Creator4/2  "vel_ref"
  Bus Creator2/1 -> Bus Creator4/1  "pose_ref"
  Selector1/1 -> Demux2/1
  Selector2/1 -> Demux3/1
  Selector3/1 -> Demux4/1
  Selector/1 -> Demux1/1
  Bus Selector/2 -> Selector1/1  "<X_ref_y>"
  Bus Selector/3 -> Selector2/1  "<X_ref_z>"
  Bus Selector/4 -> Selector3/1  "<X_ref_yaw>"
  Bus Selector/1 -> Selector/1  "<X_ref_x>"
  X_ref/1 -> Bus Selector/1

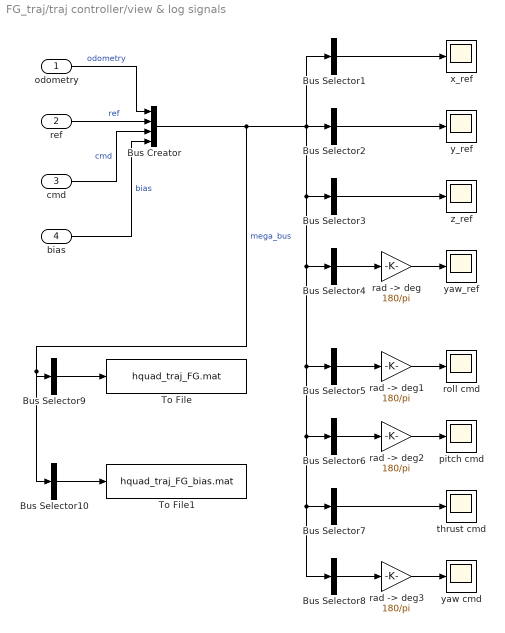
== system FG_traj/traj controller/view & log signals ==
  odometry : Inport
  ref : Inport  Port=2
  cmd : Inport  Port=3
  bias : Inport  Port=4
  Bus Creator : BusCreator
  Bus Selector1 : BusSelector  OutputSignals=odometry.pos.x,odometry.vel.x_dot,ref.pose_ref.x_ref,ref.vel_ref.x_dot_ref  OutputAsBus=on
  Bus Selector10 : BusSelector  OutputSignals=bias.pitch_bias,bias.roll_bias,bias.thrust_bias,bias.yaw_rate_bias  OutputAsBus=on
  Bus Selector2 : BusSelector  OutputSignals=odometry.pos.y,odometry.vel.y_dot,ref.pose_ref.y_ref,ref.vel_ref.y_dot_ref  OutputAsBus=on
  Bus Selector3 : BusSelector  OutputSignals=odometry.pos.z,odometry.vel.z_dot,ref.pose_ref.z_ref,ref.vel_ref.z_dot_ref  OutputAsBus=on
  Bus Selector4 : BusSelector  OutputSignals=odometry.rpy.yaw,odometry.ang_vel.ang_vel_z,ref.pose_ref.yaw_ref,ref.vel_ref.yaw_dot_ref  OutputAsBus=on
  Bus Selector5 : BusSelector  OutputSignals=odometry.rpy.roll,odometry.ang_vel.ang_vel_x,cmd.roll_cmd  OutputAsBus=on
  Bus Selector6 : BusSelector  OutputSignals=odometry.rpy.pitch,odometry.ang_vel.ang_vel_y,cmd.pitch_cmd  OutputAsBus=on
  Bus Selector7 : BusSelector  OutputSignals=odometry.pos.z,ref.pose_ref.z_ref,cmd.thrust_cmd  OutputAsBus=on
  Bus Selector8 : BusSelector  OutputSignals=odometry.rpy.yaw,odometry.ang_vel.ang_vel_z,cmd.yaw_rate_cmd  OutputAsBus=on
  Bus Selector9 : BusSelector  OutputSignals=odometry.pos.x,odometry.vel.x_dot,odometry.rpy.pitch,ref.pose_ref.x_ref,cmd.pitch_cmd,odometry.pos.y,odometry.vel.y_dot,odometry.rpy.roll,ref.pose_ref.y_ref,cmd.roll_cmd,odometry.pos.z,odometry.vel.z_dot,ref.pose_ref.z_ref,cmd.thrust_cmd,odometry.rpy.yaw,odometry.ang_vel.ang_vel_z,ref.pose_ref.yaw_ref,cmd.yaw_rate_cmd  OutputAsBus=on
  To File : ToFile  Filename=hquad_traj_FG.mat  MatrixName=hquad_traj_FG
  To File1 : ToFile  Filename=hquad_traj_FG_bias.mat  MatrixName=hquad_traj_FG_bias
  pitch cmd : Scope
      settings: YMin=-15  YMax=15  SaveName=ScopeData2
  rad -> deg{,1..3} (4 alike) : Gain  Gain=180/pi
  roll cmd : Scope
      settings: YMin=-100  YMax=100
  thrust cmd : Scope
      settings: YMin=-3  YMax=3  SaveName=ScopeData11
  x_ref : Scope
      settings: TimeRange=40  YMin=-1.5  YMax=1.5  SaveName=ScopeData3
  y_ref : Scope
      settings: TimeRange=40  YMin=-0.75  YMax=2.75
  yaw cmd : Scope
      settings: YMin=-60  YMax=-0  SaveName=ScopeData10
  yaw_ref : Scope
      settings: TimeRange=39.996  YMin=-1.5  YMax=8.5  SaveName=ScopeData8
  z_ref : Scope
      settings: TimeRange=40  YMin=-21  YMax=1  SaveName=ScopeData5
  wires:
  Bus Selector10/1 -> To File1/1
  bias/1 -> Bus Creator/4  "bias"
  Bus Selector8/1 -> "rad -> deg3"/1
  Bus Selector6/1 -> "rad -> deg2"/1
  Bus Selector5/1 -> "rad -> deg1"/1
  Bus Selector7/1 -> thrust cmd/1
  Bus Selector4/1 -> "rad -> deg"/1
  Bus Selector3/1 -> z_ref/1
  Bus Selector2/1 -> y_ref/1
  Bus Selector1/1 -> x_ref/1
  Bus Creator/1 -> Bus Selector10/1, Bus Selector9/1, Bus Selector8/1, Bus Selector7/1, Bus Selector6/1, Bus Selector5/1, Bus Selector4/1, Bus Selector3/1, Bus Selector2/1, Bus Selector1/1  "mega_bus"
  cmd/1 -> Bus Creator/3  "cmd"
  ref/1 -> Bus Creator/2  "ref"
  odometry/1 -> Bus Creator/1  "odometry"
  "rad -> deg3"/1 -> yaw cmd/1
  "rad -> deg2"/1 -> pitch cmd/1
  "rad -> deg1"/1 -> roll cmd/1
  "rad -> deg"/1 -> yaw_ref/1
  Bus Selector9/1 -> To File/1

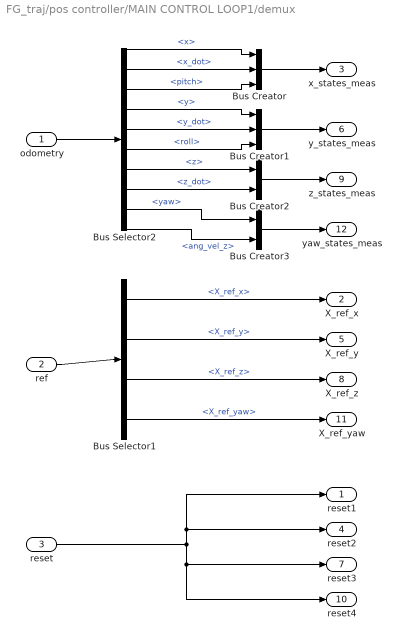
== system FG_traj/pos controller/MAIN CONTROL LOOP1/demux ==
  odometry : Inport
  ref : Inport  Port=2
  reset : Inport  Port=3
  Bus Creator : BusCreator  Inputs=3
  Bus Creator1 : BusCreator  Inputs=3
  Bus Creator2 : BusCreator  Inputs=2
  Bus Creator3 : BusCreator  Inputs=2
  Bus Selector1 : BusSelector  OutputSignals=X_ref_x,X_ref_y,X_ref_z,X_ref_yaw
  Bus Selector2 : BusSelector  OutputSignals=pos.x,vel.x_dot,rpy.pitch,pos.y,vel.y_dot,rpy.roll,pos.z,vel.z_dot,rpy.yaw,ang_vel.ang_vel_z
  reset1 : Outport
  X_ref_x : Outport  Port=2
  x_states_meas : Outport  Port=3  PortDimensions=3
  reset2 : Outport  Port=4
  X_ref_y : Outport  Port=5
  y_states_meas : Outport  Port=6  PortDimensions=3
  reset3 : Outport  Port=7
  X_ref_z : Outport  Port=8
  z_states_meas : Outport  Port=9  PortDimensions=2
  reset4 : Outport  Port=10
  X_ref_yaw : Outport  Port=11
  yaw_states_meas : Outport  Port=12  PortDimensions=2
  wires:
  Bus Selector1/4 -> X_ref_yaw/1  "<X_ref_yaw>"
  Bus Selector1/3 -> X_ref_z/1  "<X_ref_z>"
  Bus Selector2/6 -> Bus Creator1/3  "<roll>"
  Bus Selector2/3 -> Bus Creator/3  "<pitch>"
  odometry/1 -> Bus Selector2/1
  Bus Creator/1 -> x_states_meas/1
  Bus Selector2/1 -> Bus Creator/1  "<x>"
  Bus Selector2/2 -> Bus Creator/2  "<x_dot>"
  Bus Selector2/4 -> Bus Creator1/1  "<y>"
  Bus Selector2/5 -> Bus Creator1/2  "<y_dot>"
  Bus Creator1/1 -> y_states_meas/1
  Bus Selector2/7 -> Bus Creator2/1  "<z>"
  Bus Selector2/8 -> Bus Creator2/2  "<z_dot>"
  Bus Selector2/9 -> Bus Creator3/1  "<yaw>"
  Bus Selector2/10 -> Bus Creator3/2  "<ang_vel_z>"
  Bus Creator2/1 -> z_states_meas/1
  Bus Creator3/1 -> yaw_states_meas/1
  ref/1 -> Bus Selector1/1
  Bus Selector1/1 -> X_ref_x/1  "<X_ref_x>"
  Bus Selector1/2 -> X_ref_y/1  "<X_ref_y>"
  reset/1 -> reset3/1, reset4/1, reset2/1, reset1/1

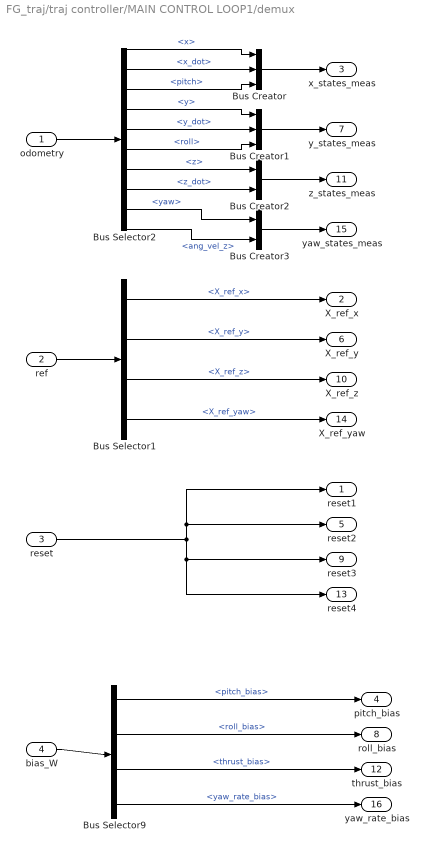
== system FG_traj/traj controller/MAIN CONTROL LOOP1/demux ==
  odometry : Inport
  ref : Inport  Port=2
  reset : Inport  Port=3
  bias_W : Inport  Port=4
  Bus Creator : BusCreator  Inputs=3
  Bus Creator1 : BusCreator  Inputs=3
  Bus Creator2 : BusCreator  Inputs=2
  Bus Creator3 : BusCreator  Inputs=2
  Bus Selector1 : BusSelector  OutputSignals=X_ref_x,X_ref_y,X_ref_z,X_ref_yaw
  Bus Selector2 : BusSelector  OutputSignals=pos.x,vel.x_dot,rpy.pitch,pos.y,vel.y_dot,rpy.roll,pos.z,vel.z_dot,rpy.yaw,ang_vel.ang_vel_z
  Bus Selector9 : BusSelector  OutputSignals=pitch_bias,roll_bias,thrust_bias,yaw_rate_bias
  reset1 : Outport
  X_ref_x : Outport  Port=2
  x_states_meas : Outport  Port=3  PortDimensions=3
  pitch_bias : Outport  Port=4
  reset2 : Outport  Port=5
  X_ref_y : Outport  Port=6
  y_states_meas : Outport  Port=7  PortDimensions=3
  roll_bias : Outport  Port=8
  reset3 : Outport  Port=9
  X_ref_z : Outport  Port=10
  z_states_meas : Outport  Port=11  PortDimensions=2
  thrust_bias : Outport  Port=12
  reset4 : Outport  Port=13
  X_ref_yaw : Outport  Port=14
  yaw_states_meas : Outport  Port=15  PortDimensions=2
  yaw_rate_bias : Outport  Port=16
  wires:
  Bus Selector9/4 -> yaw_rate_bias/1  "<yaw_rate_bias>"
  Bus Selector9/3 -> thrust_bias/1  "<thrust_bias>"
  Bus Selector9/2 -> roll_bias/1  "<roll_bias>"
  Bus Selector9/1 -> pitch_bias/1  "<pitch_bias>"
  bias_W/1 -> Bus Selector9/1
  Bus Selector1/4 -> X_ref_yaw/1  "<X_ref_yaw>"
  Bus Selector1/3 -> X_ref_z/1  "<X_ref_z>"
  Bus Selector2/6 -> Bus Creator1/3  "<roll>"
  Bus Selector2/3 -> Bus Creator/3  "<pitch>"
  odometry/1 -> Bus Selector2/1
  Bus Creator/1 -> x_states_meas/1
  Bus Selector2/1 -> Bus Creator/1  "<x>"
  Bus Selector2/2 -> Bus Creator/2  "<x_dot>"
  Bus Selector2/4 -> Bus Creator1/1  "<y>"
  Bus Selector2/5 -> Bus Creator1/2  "<y_dot>"
  Bus Creator1/1 -> y_states_meas/1
  Bus Selector2/7 -> Bus Creator2/1  "<z>"
  Bus Selector2/8 -> Bus Creator2/2  "<z_dot>"
  Bus Selector2/9 -> Bus Creator3/1  "<yaw>"
  Bus Selector2/10 -> Bus Creator3/2  "<ang_vel_z>"
  Bus Creator2/1 -> z_states_meas/1
  Bus Creator3/1 -> yaw_states_meas/1
  ref/1 -> Bus Selector1/1
  Bus Selector1/1 -> X_ref_x/1  "<X_ref_x>"
  Bus Selector1/2 -> X_ref_y/1  "<X_ref_y>"
  reset/1 -> reset3/1, reset4/1, reset2/1, reset1/1
